simulink model "piControler"  (R2016b)
settings: Solver=ode4  StartTime=0.0  StopTime=1000  FixedStep=0.002  RelTol=1e-3
values from neighbouring files (symbols this model uses):
  ac = 370.96 / fator    (= 6.18266666667)    [carregaDadosDoModelo.m]
settings Model: Creator=maripimentel  LastModifiedBy=maripimentel

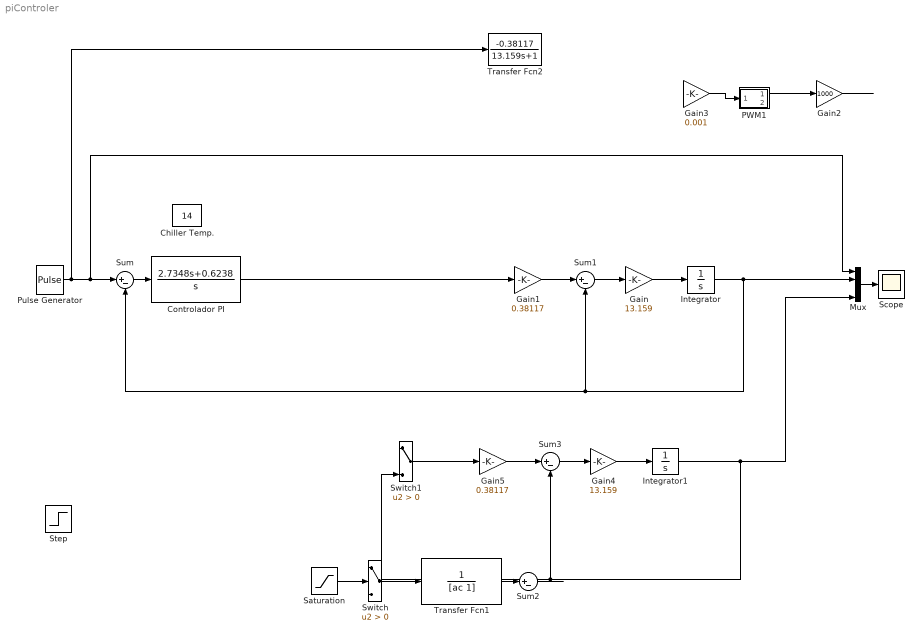
== system piControler ==
  Chiller Temp. : Constant  Value=14
  Controlador PI : TransferFcn  Numerator=[2.7348, 0.6238]  Denominator=[1,0]
  Gain : Gain  Gain=13.159
  Gain1 : Gain  Gain=0.38117
  Gain2 : Gain  Gain=1000
  Gain3 : Gain  Gain=0.001
  Gain4 : Gain  Gain=13.159
  Gain5 : Gain  Gain=0.38117
  Integrator : Integrator  InitialCondition=30
  Integrator1 : Integrator  InitialCondition=30
  Mux : Mux
  PWM1 : Subsystem  mask(Pulse Generator){period=400, amplitude=1, start=0}
      mask prompts: period "Period (secs):"; start "Start time:"
      mask help: Pulse Generator
      mask Help: Pulse generator which ensures pulse transitions are hit. Provides a vector of pulses when the height is entered as a vector.  Unmask to see how it works.
      mask Display: plot(0,0,100,100,[95,90,90,75,75,60,60,45,45,30,30,15,15,5],[25,25,75,75,25,25,75,75,25,25,75,75,25,25]);
  Pulse Generator : DiscretePulseGenerator  PulseType=Time based  Amplitude=21  Period=240  PulseWidth=75
  Saturation : Saturate  UpperLimit=1  LowerLimit=0
  Scope : Scope
  Step : Step  After=21  SampleTime=0
  Sum{,1..3} (4 alike) : Sum  Inputs=|+-
  Switch : Switch  Criteria=u2 > Threshold
  Switch1 : Switch  Criteria=u2 > Threshold
  Transfer Fcn1 : TransferFcn  Denominator=[ac 1]
  Transfer Fcn2 : TransferFcn  Numerator=[-0.38117]  Denominator=[13.159, 1]
  wires:
  Sum/1 -> Controlador PI/1
  Mux/1 -> Scope/1
  Integrator/1 -> Mux/2, Sum1/2, Sum/2
  Gain/1 -> Integrator/1
  Sum1/1 -> Gain/1
  Gain1/1 -> Sum1/1
  PWM1/1(Out1) -> Gain2/1
  Gain2/1 -> ?
  Gain3/1 -> PWM1/1(In1)
  Controlador PI/1 -> Gain1/1
  Integrator1/1 -> Switch1/3, Sum3/2, Mux/4
  Gain4/1 -> Integrator1/1
  Sum3/1 -> Gain4/1
  Gain5/1 -> Sum3/1
  Pulse Generator/1 -> Sum/1, Mux/1, Transfer Fcn2/1
  Switch1/1 -> Gain5/1
  ? -> Sum2/2
  ? -> Switch/3
  Transfer Fcn1/1 -> Sum2/1
  Sum2/1 -> ?
  Saturation/1 -> Switch/2
  Switch/1 -> Transfer Fcn1/1
  ? -> Switch/1

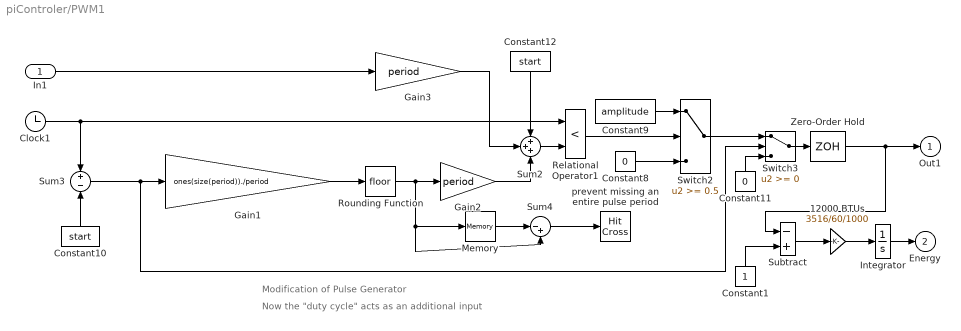
== system piControler/PWM1 ==
  note: Now the "duty cycle" acts as an additional input
  note: Modification of Pulse Generator
  In1 : Inport
  12000 BTUs : Gain  Gain=3516/60/1000
  Clock1 : Clock
  Constant1 : Constant
  Constant10 : Constant  Value=start
  Constant11 : Constant  Value=0
  Constant12 : Constant  Value=start
  Constant8 : Constant  Value=0
  Constant9 : Constant  Value=amplitude
  Gain1 : Gain  Gain=ones(size(period))./period  SaturateOnIntegerOverflow=on  OutDataTypeStr=Inherit: Same as input  ParamDataTypeStr=Inherit: Same as input
  Gain2 : Gain  Gain=period  SaturateOnIntegerOverflow=on  OutDataTypeStr=Inherit: Same as input  ParamDataTypeStr=Inherit: Same as input
  Gain3 : Gain  Gain=period  SaturateOnIntegerOverflow=on  OutDataTypeStr=Inherit: Same as input  ParamDataTypeStr=Inherit: Same as input
  Integrator : Integrator
  Memory : Memory
  Relational Operator1 : RelationalOperator  Operator=<  RndMeth=Nearest  InputSameDT=on
  Rounding Function : Rounding
  Subtract : Sum  Inputs=-+
  Sum2 : Sum  Inputs=+++  SaturateOnIntegerOverflow=on  InputSameDT=on  OutDataTypeStr=Inherit: Same as first input
  Sum3 : Sum  Inputs=+-  SaturateOnIntegerOverflow=on  InputSameDT=on  OutDataTypeStr=Inherit: Same as first input
  Sum4 : Sum  Inputs=|-+  SaturateOnIntegerOverflow=on  InputSameDT=on  OutDataTypeStr=Inherit: Same as first input
  Switch2 : Switch  Threshold=0.5  SaturateOnIntegerOverflow=on  InputSameDT=on
  Switch3 : Switch  SaturateOnIntegerOverflow=on  InputSameDT=on
  Zero-Order Hold : ZeroOrderHold  SampleTime=.1
  prevent missing an entire pulse period : HitCross  HitCrossingOffset=1  ShowOutputPort=off
  Out1 : Outport
  Energy : Outport  Port=2
  wires:
  Gain3/1 -> Sum2/2
  Constant12/1 -> Sum2/1
  In1/1 -> Gain3/1
  Gain2/1 -> Sum2/3
  Constant10/1 -> Sum3/2
  Sum3/1 -> Gain1/1, Switch3/2
  Clock1/1 -> Relational Operator1/1, Sum3/1
  Sum2/1 -> Relational Operator1/2
  Gain1/1 -> Rounding Function/1
  Rounding Function/1 -> Sum4/2, Memory/1, Gain2/1
  Switch3/1 -> Zero-Order Hold/1
  Relational Operator1/1 -> Switch2/2
  Constant8/1 -> Switch2/3
  Constant9/1 -> Switch2/1
  Constant11/1 -> Switch3/3
  Switch2/1 -> Switch3/1
  Sum4/1 -> prevent missing an entire pulse period/1
  Memory/1 -> Sum4/1
  Zero-Order Hold/1 -> Out1/1, Subtract/1
  Integrator/1 -> Energy/1
  Constant1/1 -> Subtract/2
  12000 BTUs/1 -> Integrator/1
  Subtract/1 -> 12000 BTUs/1
